simulink model "gm_wlanhdlTimeAndFrequencySynchronization"  (R2025a)
settings: Solver=FixedStepDiscrete  StartTime=0.0  StopTime=stopTime  RelTol=1e-3
InitFcn:
  | wlanFrontEndInit;
undefined symbols (not defined in the file or in its folder): a, b, c, Hd, wlanConfig
libraries: simulink x95, hdlsllib x16, hdlmdlgenlib x12, dspsrcs4 x3, dspsigops x3, dsphdlsigops2 x2, dsphdlfiltering2 x2
(part 1 of 11)
settings Model: Creator=The MathWorks, Inc.  LastModifiedBy=amd
settings SolverCC: MaxZcPerStep=1.0
settings OptimizationCC: BlockReduction=off  ConditionallyExecuteInputs=off  DefaultParameterBehavior=Inlined  ReuseModelBlockBuffer=off
settings DebuggingCC: AlgebraicLoopMsg=error  SaveWithParameterizedLinksMsg=none  InheritedTsInSrcMsg=none  SingleTaskRateTransMsg=error  UnconnectedInputMsg=warning  UnconnectedOutputMsg=warning  UnconnectedLineMsg=warning
settings HardwareCC: ProdBitPerPointer=32.0  ProdBitPerSizeT=32.0  ProdBitPerPtrDiffT=32.0  ProdLargestAtomicFloat=None  ProdIntDivRoundTo=Undefined  ProdEndianess=Unspecified  ProdWordSize=32.0  ProdHWDeviceType=ASIC/FPGA->ASIC/FPGA  TargetBitPerLong=64.0  TargetBitPerPointer=64.0  TargetBitPerSizeT=64.0  TargetBitPerPtrDiffT=64.0  TargetLongLongMode=on  TargetIntDivRoundTo=Zero  TargetEndianess=LittleEndian  TargetWordSize=64.0  TargetHWDeviceType=Custom Processor->MATLAB Host Computer  ProdEqTarget=off
settings ModelReferenceCC: EnableRefExpFcnMdlSchedulingChecks=on
settings RTWCC: GPUComputeCapability=3.5  DLArmComputeVersion=19.05

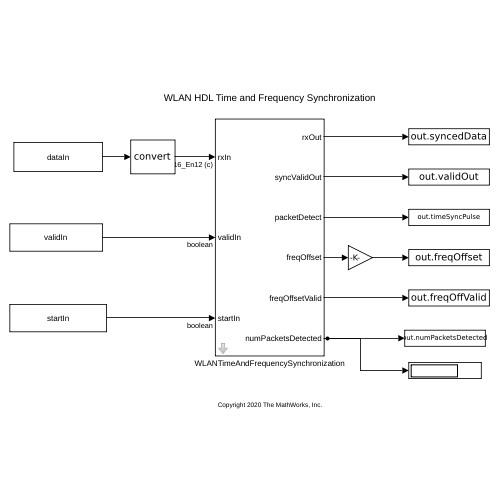
[thumbnail: Simulink's stored preview of the top-level diagram]
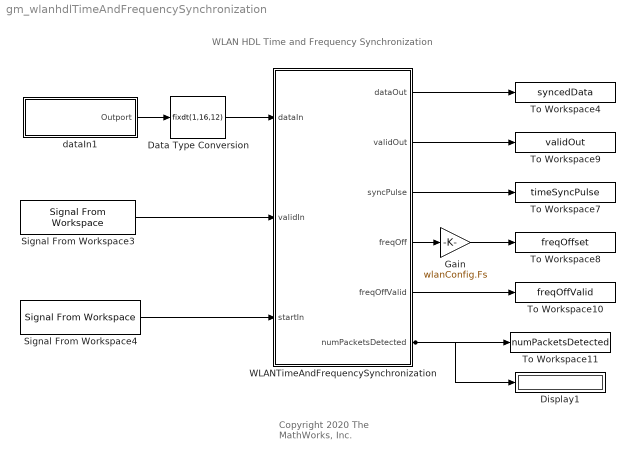
== system gm_wlanhdlTimeAndFrequencySynchronization ==
  note: WLAN HDL Time and Frequency Synchronization
  note: Copyright 2020 The MathWorks, Inc.
  Data Type Conversion : DataTypeConversion  OutDataTypeStr=fixdt(1,16,12)  SaturateOnIntegerOverflow=off  RndMeth=Floor
  Display1 : Display
  Gain : Gain  Gain=wlanConfig.Fs
  Signal From Workspace3 : dspsrcs4/Signal From Workspace  X=validIn  Ts=1/wlanConfig.Fs  nsamps=1  OutputAfterFinalValue=Setting to zero  ignoreOrWarnInputAndFrameLengths=off  OutputFrames=off
  Signal From Workspace4 : dspsrcs4/Signal From Workspace  X=startIn  Ts=1/wlanConfig.Fs  nsamps=1  OutputAfterFinalValue=Setting to zero  ignoreOrWarnInputAndFrameLengths=off  OutputFrames=off
  To Workspace10 : ToWorkspace  VariableName=freqOffValid  SampleTime=-1
      settings: Save2DSignal=2-D array (concatenate along first dimension)
  To Workspace11 : ToWorkspace  VariableName=numPacketsDetected  SampleTime=-1
      settings: Save2DSignal=2-D array (concatenate along first dimension)
  To Workspace4 : ToWorkspace  VariableName=syncedData  SampleTime=-1
      settings: Save2DSignal=2-D array (concatenate along first dimension)
  To Workspace7 : ToWorkspace  VariableName=timeSyncPulse  SampleTime=-1
      settings: Save2DSignal=2-D array (concatenate along first dimension)
  To Workspace8 : ToWorkspace  VariableName=freqOffset  SampleTime=-1
      settings: Save2DSignal=2-D array (concatenate along first dimension)
  To Workspace9 : ToWorkspace  VariableName=validOut  SampleTime=-1
      settings: Save2DSignal=2-D array (concatenate along first dimension)
  WLANTimeAndFrequencySynchronization : Subsystem  mask(WLAN Front end application){chanBW=20MHz}
      mask prompts: chanBW "Channel bandwidth:"
      mask help: Performs time and frequency synchronization.
      mask Help: eval('showExample(''whdl/WLANHDLTimeAndFrequencySynchronizationExample'')')
      mask TypeOptions chanBW: 20MHz | 40MHz | 80MHz
      mask Display:
      | port_label('input',1,'rxIn');
      | port_label('input',2,'validIn');
      | port_label('input',3,'startIn');
      | port_label('output',1,'rxOut');
      | port_label('output',2,'syncValidOut');
      | port_label('output',3,'packetDetect');
      | port_label('output',4,'freqOffset');
      | port_label('output',5,'freqOffsetValid');
      | 
      | port_label('output',6,'numPacketsDetected');
  dataIn1 : Subsystem
      mask Display: disp('dataIn');
  wires:
  Gain/1 -> To Workspace8/1
  WLANTimeAndFrequencySynchronization/4(freqOff) -> Gain/1
  dataIn1/1(Outport) -> Data Type Conversion/1
  Data Type Conversion/1 -> WLANTimeAndFrequencySynchronization/1(dataIn)
  WLANTimeAndFrequencySynchronization/1(dataOut) -> To Workspace4/1
  WLANTimeAndFrequencySynchronization/2(validOut) -> To Workspace9/1
  Signal From Workspace4/1 -> WLANTimeAndFrequencySynchronization/3(startIn)
  WLANTimeAndFrequencySynchronization/3(syncPulse) -> To Workspace7/1
  WLANTimeAndFrequencySynchronization/6(numPacketsDetected) -> Display1/1, To Workspace11/1
  WLANTimeAndFrequencySynchronization/5(freqOffValid) -> To Workspace10/1
  Signal From Workspace3/1 -> WLANTimeAndFrequencySynchronization/2(validIn)

== system gm_wlanhdlTimeAndFrequencySynchronization/WLANTimeAndFrequencySynchronization ==
  dataIn : Inport  OutDataTypeStr=fixdt(1, 16, 12)  PortDimensions=1  SampleTime=5e-08
      settings: SignalType=complex
  validIn : Inport  Port=2  OutDataTypeStr=boolean  PortDimensions=1  SampleTime=5e-08
  startIn : Inport  Port=3  OutDataTypeStr=boolean  PortDimensions=1  SampleTime=5e-08
  Add : Sum  OutDataTypeStr=fixdt(1, 35, 33)  AccumDataTypeStr=fixdt(1, 35, 33)  SampleTime=6.25e-09
  Coarse CFO Estimation and Correction : Subsystem
  Coarse Time Sync : Subsystem
  Delay1 : Delay  DelayLength=double(1)  InitialCondition=0  SampleTime=5e-08
  Delay2 : Delay  DelayLength=double(1)  InitialCondition=0  SampleTime=5e-08
  Delay3 : Delay  DelayLength=double(1)  InitialCondition=0  SampleTime=5e-08
  Fine CFO Estimation and Correction : Subsystem
  Fine Time Sync : Subsystem
  HDL Counter : RateTransition  InitialCondition=double(0)  OutPortSampleTimeOpt=Multiple of input port sample time  OutPortSampleTimeMultiple=8
  HDL Counter_absorbed : Delay  DelayLength=0
  Rx Filter : Subsystem
  adder : Sum  OutDataTypeStr=uint16  AccumDataTypeStr=uint16  SampleTime=6.25e-09
  compare : simulink/Logic and Bit Operations/Compare To Constant  relop===  const="fi(0,0,16,0,\"hex\",\"ffff\")"  OutDataTypeStr=boolean
  countFrom : Constant  Value=0  VectorParams1D=off  OutDataTypeStr=uint16  SampleTime=6.25e-09
  crp_out_delay : Delay  DelayLength=double(1)  InitialCondition=0  SampleTime=6.25e-09
  in0_repeat : RateTransition  Integrity=off  Deterministic=off  OutPortSampleTimeOpt=Multiple of input port sample time  OutPortSampleTimeMultiple=1/8
  in1_repeat : RateTransition  Integrity=off  Deterministic=off  OutPortSampleTimeOpt=Multiple of input port sample time  OutPortSampleTimeMultiple=1/8
  in2_repeat : RateTransition  Integrity=off  Deterministic=off  OutPortSampleTimeOpt=Multiple of input port sample time  OutPortSampleTimeMultiple=1/8
  in3_repeat : RateTransition  Integrity=off  Deterministic=off  OutPortSampleTimeOpt=Multiple of input port sample time  OutPortSampleTimeMultiple=1/8
  rd_{0,3..5} (4 alike) : Delay  DelayLength=double(1)  InitialCondition=0  SampleTime=6.25e-09
  rd_1 : Delay  DelayLength=double(3)  InitialCondition=0  SampleTime=6.25e-09
  rd_2 : Delay  DelayLength=double(2)  InitialCondition=0  SampleTime=6.25e-09
  step_value : Constant  VectorParams1D=off  OutDataTypeStr=uint16  SampleTime=6.25e-09
  switch : Switch  Criteria=u2 ~= 0  Threshold="fi(0,0,1,0,\"hex\",\"0\")"  OutDataTypeStr=uint16  SampleTime=6.25e-09  SaturateOnIntegerOverflow=off  InputSameDT=off
  switchEnable : MultiPortSwitch  DataPortOrder=Zero-based contiguous  Inputs=2  DiagnosticForDefault=None  zeroidx=on  OutDataTypeStr=uint16  SampleTime=6.25e-09  SaturateOnIntegerOverflow=off  InputSameDT=off
  t : RateTransition  InitialCondition=double(0)  OutPortSampleTimeOpt=Multiple of input port sample time  OutPortSampleTimeMultiple=8
  dataOut : Outport  SampleTime=5e-08
  validOut : Outport  Port=2  SampleTime=5e-08
  syncPulse : Outport  Port=3  SampleTime=5e-08
  freqOff : Outport  Port=4  SampleTime=5e-08
  freqOffValid : Outport  Port=5  SampleTime=5e-08
  numPacketsDetected : Outport  Port=6  SampleTime=5e-08
  wires:
  rd_5/1 -> switchEnable/3
  countFrom/1 -> switch/1
  compare/1 -> rd_3/1
  in1_repeat/1 -> rd_0/1
  rd_4/1 -> switch/3
  step_value/1 -> adder/2
  HDL Counter/1 -> HDL Counter_absorbed/1
  crp_out_delay/1 -> HDL Counter/1
  switchEnable/1 -> crp_out_delay/1
  t/1 -> freqOff/1
  rd_1/1 -> switchEnable/1
  rd_2/1 -> switchEnable/2
  in0_repeat/1 -> rd_1/1
  Coarse Time Sync/4(rst) -> Coarse CFO Estimation and Correction/4(rstIn)
  HDL Counter_absorbed/1 -> in1_repeat/1, numPacketsDetected/1
  Rx Filter/2(validOut) -> Coarse Time Sync/2(validIn)
  rd_0/1 -> rd_2/1, compare/1, adder/1
  Coarse CFO Estimation and Correction/3(validOut) -> Fine Time Sync/2(validIn)
  Add/1 -> t/1
  Delay1/1 -> Rx Filter/3(startIn)
  in2_repeat/1 -> Add/1
  Delay2/1 -> Rx Filter/2(validIn)
  Rx Filter/3(startOut) -> Coarse Time Sync/3(startIn)
  startIn/1 -> Delay1/1
  Coarse CFO Estimation and Correction/4(lstfStartOut) -> Fine Time Sync/3(lstfStart)
  validIn/1 -> Delay2/1
  Coarse Time Sync/2(validOut) -> Coarse CFO Estimation and Correction/2(validIn)
  Fine CFO Estimation and Correction/5(lstfStartOut) -> in0_repeat/1, syncPulse/1
  adder/1 -> rd_4/1
  Rx Filter/1(dataOut) -> Coarse Time Sync/1(dataIn)
  in3_repeat/1 -> Add/2
  Delay3/1 -> Rx Filter/1(dataIn)
  Fine Time Sync/2(validOut) -> Fine CFO Estimation and Correction/2(validIn)
  Coarse Time Sync/3(lstfStart) -> Coarse CFO Estimation and Correction/3(LSTF_start)
  dataIn/1 -> Delay3/1
  Coarse CFO Estimation and Correction/1(Freq) -> in2_repeat/1
  Coarse CFO Estimation and Correction/2(dataOut) -> Fine Time Sync/1(dataIn)
  switch/1 -> rd_5/1
  rd_3/1 -> switch/2
  Coarse Time Sync/1(dataOut) -> Coarse CFO Estimation and Correction/1(dataIn)
  Coarse CFO Estimation and Correction/5(rstOut) -> Fine Time Sync/4(rstIn)
  Fine CFO Estimation and Correction/1(Freq) -> in3_repeat/1
  Fine Time Sync/3(Lstf_start) -> Fine CFO Estimation and Correction/3(LSTF_start)
  Fine CFO Estimation and Correction/2(freqValidOut) -> freqOffValid/1
  Fine Time Sync/4(rstOut) -> Fine CFO Estimation and Correction/4(rstIn)
  Fine Time Sync/1(dataOut) -> Fine CFO Estimation and Correction/1(dataIn)
  Fine CFO Estimation and Correction/3(dataOut) -> dataOut/1
  Fine CFO Estimation and Correction/4(validOut) -> validOut/1

== system gm_wlanhdlTimeAndFrequencySynchronization/dataIn1 ==
  Signal From Workspace : dspsrcs4/Signal From Workspace  X=inputWaveform  Ts=1/wlanConfig.Fs  nsamps=1  OutputAfterFinalValue=Setting to zero  ignoreOrWarnInputAndFrameLengths=off  OutputFrames=off
  Outport : Outport
  wires:
  Signal From Workspace/1 -> Outport/1

== system gm_wlanhdlTimeAndFrequencySynchronization/WLANTimeAndFrequencySynchronization/Coarse CFO Estimation and Correction ==
  dataIn : Inport  OutDataTypeStr=fixdt(1, 16, 12)  PortDimensions=1  SampleTime=5e-08
      settings: SignalType=complex
  validIn : Inport  Port=2  OutDataTypeStr=boolean  PortDimensions=1  SampleTime=6.25e-09
  LSTF_start : Inport  Port=3  OutDataTypeStr=boolean  PortDimensions=1  SampleTime=6.25e-09
  rstIn : Inport  Port=4  OutDataTypeStr=boolean  PortDimensions=1  SampleTime=5e-08
  Coarse CFO Correction : Subsystem
  Coarse CFO Estimation : Subsystem
  Freq : Outport  SampleTime=5e-08
  dataOut : Outport  Port=2  SampleTime=5e-08
  validOut : Outport  Port=3  SampleTime=5e-08
  lstfStartOut : Outport  Port=4  SampleTime=5e-08
  rstOut : Outport  Port=5  SampleTime=5e-08
  wires:
  Coarse CFO Correction/5(rstOut) -> rstOut/1
  dataIn/1 -> Coarse CFO Estimation/1(dataIn)
  Coarse CFO Estimation/4(lstfStart) -> Coarse CFO Correction/4(lstfStartIn)
  validIn/1 -> Coarse CFO Estimation/2(validIn)
  rstIn/1 -> Coarse CFO Estimation/4(rstIn)
  Coarse CFO Correction/1(freqOut) -> Freq/1
  Coarse CFO Correction/2(dataOut) -> dataOut/1
  Coarse CFO Estimation/2(dataOut) -> Coarse CFO Correction/2(dataIn)
  Coarse CFO Estimation/3(validData) -> Coarse CFO Correction/3(validIn)
  LSTF_start/1 -> Coarse CFO Estimation/3(LSTF_start)
  Coarse CFO Correction/4(lstfStartOut) -> lstfStartOut/1
  Coarse CFO Estimation/5(rstOut) -> Coarse CFO Correction/5(rstIn)
  Coarse CFO Estimation/1(Freq) -> Coarse CFO Correction/1(freq)
  Coarse CFO Correction/3(validOut) -> validOut/1

== system gm_wlanhdlTimeAndFrequencySynchronization/WLANTimeAndFrequencySynchronization/Coarse Time Sync ==
  dataIn : Inport  OutDataTypeStr=fixdt(1, 16, 12)  PortDimensions=1  SampleTime=5e-08
      settings: SignalType=complex
  validIn : Inport  Port=2  OutDataTypeStr=boolean  PortDimensions=1  SampleTime=5e-08
  startIn : Inport  Port=3  OutDataTypeStr=boolean  PortDimensions=1  SampleTime=5e-08
  Correlator : Subsystem
  Delay4 : Delay  DelayLength=double(7)  InitialCondition=0  SampleTime=5e-08
  Delay6 : Delay  DelayLength=double(7)  InitialCondition=0  SampleTime=5e-08
  Energy Calculator : Subsystem
  Peak Detector : Subsystem
  Stream Synchronizer : Subsystem
  dataOut : Outport  SampleTime=5e-08  VectorParamsAs1DForOutWhenUnconnected=off
  validOut : Outport  Port=2  SampleTime=6.25e-09  VectorParamsAs1DForOutWhenUnconnected=off
  lstfStart : Outport  Port=3  SampleTime=6.25e-09  VectorParamsAs1DForOutWhenUnconnected=off
  rst : Outport  Port=4  SampleTime=5e-08  VectorParamsAs1DForOutWhenUnconnected=off
  wires:
  Peak Detector/2(validOut) -> validOut/1
  startIn/1 -> rst/1, Correlator/3(startIn)
  dataIn/1 -> Delay4/1, Energy Calculator/3(dataIn), Correlator/1(dataIn)
  validIn/1 -> Delay6/1, Correlator/2(validIn), Energy Calculator/4(validIn)
  Correlator/1(dataOut) -> Energy Calculator/1(corrIn)
  Correlator/2(validOut) -> Stream Synchronizer/1(corrValid), Energy Calculator/2(corrValidIn)
  Delay4/1 -> Stream Synchronizer/2(dataIn)
  Stream Synchronizer/1(dataOut) -> Peak Detector/4(dataIn)
  Peak Detector/1(lstfStart) -> lstfStart/1
  Delay6/1 -> Stream Synchronizer/3(dataValid)
  Peak Detector/3(dataOut) -> dataOut/1
  Energy Calculator/2(energyOut) -> Peak Detector/2(energyIn)
  Energy Calculator/3(validOut) -> Peak Detector/3(corrValid)
  Energy Calculator/1(corrOut) -> Peak Detector/1(corrIn)
  Stream Synchronizer/2(validOut) -> Peak Detector/5(dataValid)

== system gm_wlanhdlTimeAndFrequencySynchronization/WLANTimeAndFrequencySynchronization/Fine CFO Estimation and Correction ==
  dataIn : Inport  OutDataTypeStr=fixdt(1, 16, 12)  PortDimensions=1  SampleTime=5e-08
      settings: SignalType=complex
  validIn : Inport  Port=2  OutDataTypeStr=boolean  PortDimensions=1  SampleTime=6.25e-09
  LSTF_start : Inport  Port=3  OutDataTypeStr=boolean  PortDimensions=1  SampleTime=6.25e-09
  rstIn : Inport  Port=4  OutDataTypeStr=boolean  PortDimensions=1  SampleTime=5e-08
  Fine CFO Correction : Subsystem
  Fine CFO Estimation : Subsystem
  Freq : Outport  SampleTime=5e-08
  freqValidOut : Outport  Port=2  SampleTime=5e-08
  dataOut : Outport  Port=3  SampleTime=5e-08
  validOut : Outport  Port=4  SampleTime=5e-08
  lstfStartOut : Outport  Port=5  SampleTime=5e-08
  wires:
  dataIn/1 -> Fine CFO Estimation/1(dataIn)
  Fine CFO Correction/3(dataOut) -> dataOut/1
  validIn/1 -> Fine CFO Estimation/2(validIn)
  rstIn/1 -> Fine CFO Estimation/4(rstIn)
  Fine CFO Correction/4(validOut) -> validOut/1
  Fine CFO Correction/5(lstfStartOut) -> lstfStartOut/1
  LSTF_start/1 -> Fine CFO Estimation/3(LSTF_start)
  Fine CFO Estimation/1(Freq) -> Fine CFO Correction/1(freqIn)
  Fine CFO Estimation/3(dataOut) -> Fine CFO Correction/3(dataIn)
  Fine CFO Estimation/4(validOut) -> Fine CFO Correction/4(validIn)
  Fine CFO Correction/1(freqOut) -> Freq/1
  Fine CFO Estimation/2(freqValidOut) -> Fine CFO Correction/2(freqValidIn)
  Fine CFO Estimation/5(lstfStart) -> Fine CFO Correction/5(lstfStartIn)
  Fine CFO Correction/2(freqValidOut) -> freqValidOut/1

== system gm_wlanhdlTimeAndFrequencySynchronization/WLANTimeAndFrequencySynchronization/Fine Time Sync ==
  dataIn : Inport  OutDataTypeStr=fixdt(1, 16, 12)  PortDimensions=1  SampleTime=5e-08
      settings: SignalType=complex
  validIn : Inport  Port=2  OutDataTypeStr=boolean  PortDimensions=1  SampleTime=5e-08
  lstfStart : Inport  Port=3  OutDataTypeStr=boolean  PortDimensions=1  SampleTime=5e-08
  rstIn : Inport  Port=4  OutDataTypeStr=boolean  PortDimensions=1  SampleTime=5e-08
  Correlator : Subsystem
  Peak Searcher : Subsystem
  dataOut : Outport  SampleTime=5e-08  VectorParamsAs1DForOutWhenUnconnected=off
  validOut : Outport  Port=2  SampleTime=6.25e-09  VectorParamsAs1DForOutWhenUnconnected=off
  Lstf_start : Outport  Port=3  SampleTime=6.25e-09  VectorParamsAs1DForOutWhenUnconnected=off
  rstOut : Outport  Port=4  SampleTime=5e-08  VectorParamsAs1DForOutWhenUnconnected=off
  wires:
  Correlator/5(validOut) -> Peak Searcher/5(validIn)
  Correlator/3(startOut) -> Peak Searcher/3(startIn)
  Correlator/2(corrValid) -> Peak Searcher/2(corrValid)
  Peak Searcher/2(validOut) -> validOut/1
  Correlator/4(dataOut) -> Peak Searcher/4(dataIn)
  Correlator/1(corrOut) -> Peak Searcher/1(corrIn)
  rstIn/1 -> rstOut/1, Correlator/4(rstIn), Peak Searcher/6(rstIn)
  Peak Searcher/1(lstfStart) -> Lstf_start/1
  lstfStart/1 -> Correlator/3(startIn)
  validIn/1 -> Correlator/2(validIn)
  Peak Searcher/3(dataOut) -> dataOut/1
  dataIn/1 -> Correlator/1(dataIn)

== system gm_wlanhdlTimeAndFrequencySynchronization/WLANTimeAndFrequencySynchronization/Rx Filter ==
  dataIn : Inport  OutDataTypeStr=fixdt(1, 16, 12)  PortDimensions=1  SampleTime=5e-08
      settings: SignalType=complex
  validIn : Inport  Port=2  OutDataTypeStr=boolean  PortDimensions=1  SampleTime=5e-08
  startIn : Inport  Port=3  OutDataTypeStr=boolean  PortDimensions=1  SampleTime=5e-08
  DTConverter : Subsystem
  Delay : Delay  DelayLength=double(33)  InitialCondition=0  SampleTime=5e-08
  Discrete FIR Filter : dsphdlfiltering2/Discrete FIR Filter  NumeratorSource=Property  Numerator=Hd.Numerator  NumeratorPrototype=[]  FilterStructure=Direct form systolic  SerializationOption=Minimum number of cycles between valid input samples  NumCycles=2  NumberOfMultipliers=2  SimulateUsing=Code generation  roundingMode=Floor  overflowMode=off  CoefficientsDataTypeStr=Inherit: Same word length as input  OutputDataTypeStr=Inherit: Same word length as input  ResetInputPort=on  HDLGlobalReset=off  CoeffMultiplier=Multiplier  UseMultForPow2Coeff=on  FrameInputSymmOptim=off
  dataOut : Outport  SampleTime=5e-08
  validOut : Outport  Port=2  SampleTime=5e-08
  startOut : Outport  Port=3  SampleTime=5e-08
  wires:
  DTConverter/1(dataOut) -> dataOut/1
  Delay/1 -> startOut/1
  Discrete FIR Filter/2 -> validOut/1
  startIn/1 -> Discrete FIR Filter/3, Delay/1
  validIn/1 -> Discrete FIR Filter/2
  Discrete FIR Filter/1 -> DTConverter/2(dataIn2)
  dataIn/1 -> Discrete FIR Filter/1, DTConverter/1(dataIn1)

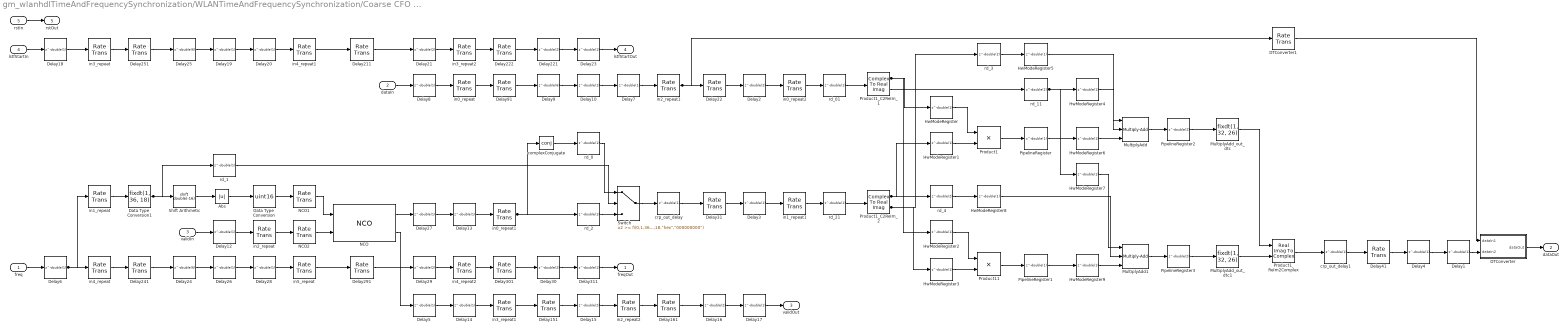
== system gm_wlanhdlTimeAndFrequencySynchronization/WLANTimeAndFrequencySynchronization/Coarse CFO Estimation and Correction/Coarse CFO Correction ==
  freq : Inport  OutDataTypeStr=fixdt(1, 34, 33)  PortDimensions=1  SampleTime=5e-08
  dataIn : Inport  Port=2  OutDataTypeStr=fixdt(1, 16, 12)  PortDimensions=1  SampleTime=5e-08
      settings: SignalType=complex
  validIn : Inport  Port=3  OutDataTypeStr=boolean  PortDimensions=1  SampleTime=5e-08
  lstfStartIn : Inport  Port=4  OutDataTypeStr=boolean  PortDimensions=1  SampleTime=5e-08
  rstIn : Inport  Port=5  OutDataTypeStr=boolean  PortDimensions=1  SampleTime=5e-08
  Abs : Abs  SampleTime=6.25e-09  OutDataTypeStr=fixdt(1, 36, 18)  SaturateOnIntegerOverflow=off
  DTConverter : Subsystem
  DTConverter1 : RateTransition  InitialCondition=double(0)  OutPortSampleTimeOpt=Multiple of input port sample time  OutPortSampleTimeMultiple=8
  Data Type  Conversion : DataTypeConversion  OutDataTypeStr=uint16  RndMeth=Round  SampleTime=6.25e-09  SaturateOnIntegerOverflow=off
  Data Type  Conversion1 : DataTypeConversion  OutDataTypeStr=fixdt(1, 36, 18)  SampleTime=6.25e-09  SaturateOnIntegerOverflow=off  RndMeth=Floor
  Delay{1,3..8,10,12..14,17..20,23,26..28,311} (20 alike) : Delay  DelayLength=double(1)  InitialCondition=0  SampleTime=5e-08
  Delay{2,15..16,21,29..30,221} (7 alike) : Delay  DelayLength=double(2)  InitialCondition=0  SampleTime=5e-08
  Delay{22,31,41,91,151,161,211,222,241,251,291,301} (12 alike) : RateTransition  InitialCondition=double(0)  OutPortSampleTimeOpt=Multiple of input port sample time  OutPortSampleTimeMultiple=8
  Delay24 : Delay  DelayLength=double(6)  InitialCondition=0  SampleTime=5e-08
  Delay25 : Delay  DelayLength=double(6)  InitialCondition=0  SampleTime=5e-08
  Delay9 : Delay  DelayLength=double(6)  InitialCondition=0  SampleTime=5e-08
  HwModeRegister{,1..9} (10 alike) : Delay  DelayLength=double(1)  InitialCondition=0  SampleTime=6.25e-09
  MultiplyAdd : hdlsllib/HDL Operations/Multiply-Add  Function=c-(a.*b)  datatype=fixdt(1, 33, 26)  DoSatur=off  FMA=off
  MultiplyAdd1 : hdlsllib/HDL Operations/Multiply-Add  Function=c+(a.*b)  datatype=fixdt(1, 33, 26)  DoSatur=off  FMA=off
  MultiplyAdd_out_dtc : DataTypeConversion  OutDataTypeStr=fixdt(1, 32, 26)  SampleTime=6.25e-09  SaturateOnIntegerOverflow=off  RndMeth=Floor
  MultiplyAdd_out_dtc1 : DataTypeConversion  OutDataTypeStr=fixdt(1, 32, 26)  SampleTime=6.25e-09  SaturateOnIntegerOverflow=off  RndMeth=Floor
  NCO : dsphdlsigops2/NCO  PhaseIncrementSource=Input port  PhaseIncrement=100  PhaseOffsetSource=Property  PhaseOffset=0  DitherSource=None  NumDitherBits=4  SamplesPerFrame=1  LUTCompress=off  ResetAction=off  Waveform=Complex exponential  PhasePort=off  SimulateUsing=Code generation  AccumulatorWL=16  PhaseQuantization=on  NumQuantizerAccumulatorBits=16  OutputDataType=Binary point scaling  OutputWL=16  OutputFL=14
  NCO1 : RateTransition  InitialCondition=double(0)  OutPortSampleTimeOpt=Multiple of input port sample time  OutPortSampleTimeMultiple=8
  NCO2 : RateTransition  InitialCondition=double(0)  OutPortSampleTimeOpt=Multiple of input port sample time  OutPortSampleTimeMultiple=8
  PipelineRegister : Delay  DelayLength=double(1)  InitialCondition=0  SampleTime=6.25e-09
  PipelineRegister1 : Delay  DelayLength=double(1)  InitialCondition=0  SampleTime=6.25e-09
  PipelineRegister2 : Delay  DelayLength=double(2)  InitialCondition=0  SampleTime=6.25e-09
  PipelineRegister3 : Delay  DelayLength=double(2)  InitialCondition=0  SampleTime=6.25e-09
  Product1 : Product  Inputs=**  OutDataTypeStr=fixdt(1, 32, 26)  SampleTime=6.25e-09
  Product11 : Product  Inputs=**  OutDataTypeStr=fixdt(1, 32, 26)  SampleTime=6.25e-09
  Product1_C2ReIm_1 : ComplexToRealImag  SampleTime=6.25e-09
  Product1_C2ReIm_2 : ComplexToRealImag  SampleTime=6.25e-09
  Product1_ReIm2Complex : RealImagToComplex  SampleTime=6.25e-09
  Shift Arithmetic : ArithShift  BitShiftNumber=double(-16)  BinPtShiftNumber=double(0)
  Switch : Switch  Threshold="fi(0,1,36,18,\"hex\",\"000000000\")"  OutDataTypeStr=fixdt(1, 16, 14)  SampleTime=6.25e-09  SaturateOnIntegerOverflow=off  InputSameDT=off
  complexConjugate : Math  Operator=conj  SignedPower=on  OutDataTypeStr=fixdt(1, 16, 14)
  crp_out_delay : Delay  DelayLength=double(1)  InitialCondition=0  SampleTime=6.25e-09
  crp_out_delay1 : Delay  DelayLength=double(1)  InitialCondition=0  SampleTime=6.25e-09
  in0_repeat : RateTransition  Integrity=off  Deterministic=off  OutPortSampleTimeOpt=Multiple of input port sample time  OutPortSampleTimeMultiple=1/8
  in0_repeat1 : RateTransition  Integrity=off  Deterministic=off  OutPortSampleTimeOpt=Multiple of input port sample time  OutPortSampleTimeMultiple=1/8
  in0_repeat2 : RateTransition  Integrity=off  Deterministic=off  OutPortSampleTimeOpt=Multiple of input port sample time  OutPortSampleTimeMultiple=1/8
  in1_repeat : RateTransition  Integrity=off  Deterministic=off  OutPortSampleTimeOpt=Multiple of input port sample time  OutPortSampleTimeMultiple=1/8
  in1_repeat1 : RateTransition  Integrity=off  Deterministic=off  OutPortSampleTimeOpt=Multiple of input port sample time  OutPortSampleTimeMultiple=1/8
  in2_repeat : RateTransition  Integrity=off  Deterministic=off  OutPortSampleTimeOpt=Multiple of input port sample time  OutPortSampleTimeMultiple=1/8
  in2_repeat1 : RateTransition  Integrity=off  Deterministic=off  OutPortSampleTimeOpt=Multiple of input port sample time  OutPortSampleTimeMultiple=1/8
  in2_repeat2 : RateTransition  Integrity=off  Deterministic=off  OutPortSampleTimeOpt=Multiple of input port sample time  OutPortSampleTimeMultiple=1/8
  in3_repeat : RateTransition  Integrity=off  Deterministic=off  OutPortSampleTimeOpt=Multiple of input port sample time  OutPortSampleTimeMultiple=1/8
  in3_repeat1 : RateTransition  Integrity=off  Deterministic=off  OutPortSampleTimeOpt=Multiple of input port sample time  OutPortSampleTimeMultiple=1/8
  in3_repeat2 : RateTransition  Integrity=off  Deterministic=off  OutPortSampleTimeOpt=Multiple of input port sample time  OutPortSampleTimeMultiple=1/8
  in4_repeat : RateTransition  Integrity=off  Deterministic=off  OutPortSampleTimeOpt=Multiple of input port sample time  OutPortSampleTimeMultiple=1/8
  in4_repeat1 : RateTransition  Integrity=off  Deterministic=off  OutPortSampleTimeOpt=Multiple of input port sample time  OutPortSampleTimeMultiple=1/8
  in4_repeat2 : RateTransition  Integrity=off  Deterministic=off  OutPortSampleTimeOpt=Multiple of input port sample time  OutPortSampleTimeMultiple=1/8
  in5_repeat : RateTransition  Integrity=off  Deterministic=off  OutPortSampleTimeOpt=Multiple of input port sample time  OutPortSampleTimeMultiple=1/8
  rd_{0..2,21} (4 alike) : Delay  DelayLength=double(1)  InitialCondition=0  SampleTime=6.25e-09
  rd_01 : Delay  DelayLength=double(1)  InitialCondition=0  SampleTime=6.25e-09
  rd_11 : Delay  DelayLength=double(2)  InitialCondition=0  SampleTime=6.25e-09
  rd_3 : Delay  DelayLength=double(2)  InitialCondition=0  SampleTime=6.25e-09
  rd_4 : Delay  DelayLength=double(2)  InitialCondition=0  SampleTime=6.25e-09
  freqOut : Outport  SampleTime=5e-08  VectorParamsAs1DForOutWhenUnconnected=off
  dataOut : Outport  Port=2  SampleTime=5e-08  VectorParamsAs1DForOutWhenUnconnected=off
  validOut : Outport  Port=3  SampleTime=5e-08  VectorParamsAs1DForOutWhenUnconnected=off
  lstfStartOut : Outport  Port=4  SampleTime=5e-08  VectorParamsAs1DForOutWhenUnconnected=off
  rstOut : Outport  Port=5  SampleTime=5e-08  VectorParamsAs1DForOutWhenUnconnected=off
  wires:
  DTConverter/1(dataOut) -> dataOut/1
  Delay41/1 -> Delay4/1
  Product1_ReIm2Complex/1 -> crp_out_delay1/1
  PipelineRegister3/1 -> MultiplyAdd_out_dtc1/1
  PipelineRegister2/1 -> MultiplyAdd_out_dtc/1
  MultiplyAdd1/1 -> PipelineRegister3/1
  MultiplyAdd/1 -> PipelineRegister2/1
  HwModeRegister4/1 -> MultiplyAdd/1
  PipelineRegister1/1 -> HwModeRegister9/1
  rd_11/1 -> HwModeRegister7/1, HwModeRegister4/1
  HwModeRegister5/1 -> MultiplyAdd/2
  HwModeRegister8/1 -> MultiplyAdd1/2
  Product1/1 -> PipelineRegister/1
  HwModeRegister2/1 -> Product11/1
  HwModeRegister1/1 -> Product1/2
  Product1_C2ReIm_2/1 -> HwModeRegister1/1, rd_4/1
  MultiplyAdd_out_dtc/1 -> Product1_ReIm2Complex/1
  Product1_C2ReIm_1/2 -> rd_11/1
  rd_21/1 -> Product1_C2ReIm_2/1
  rd_01/1 -> Product1_C2ReIm_1/1
  Delay17/1 -> validOut/1
  Delay3/1 -> in1_repeat1/1
  Delay2/1 -> in0_repeat2/1
  Delay16/1 -> Delay17/1
  Delay31/1 -> Delay3/1
  HwModeRegister/1 -> Product1/1
  Product1_C2ReIm_2/2 -> HwModeRegister3/1, rd_3/1
  crp_out_delay/1 -> Delay31/1
  Product11/1 -> PipelineRegister1/1
  in2_repeat1/1 -> Delay22/1, DTConverter1/1
  crp_out_delay1/1 -> Delay41/1
  Switch/1 -> crp_out_delay/1
  Delay211/1 -> Delay21/1
  Delay22/1 -> Delay2/1
  in3_repeat/1 -> Delay251/1
  Delay28/1 -> in5_repeat/1
  Delay12/1 -> in2_repeat/1
  rd_1/1 -> Switch/2
  Delay251/1 -> Delay25/1
  Data Type  Conversion1/1 -> Shift Arithmetic/1, rd_1/1
  in2_repeat2/1 -> Delay161/1
  Delay311/1 -> freqOut/1
  NCO1/1 -> NCO/1
  in2_repeat/1 -> NCO2/1
  DTConverter1/1 -> DTConverter/1(dataIn1)
  Delay19/1 -> Delay20/1
  in1_repeat1/1 -> rd_21/1
  in0_repeat2/1 -> rd_01/1
  Abs/1 -> Data Type  Conversion/1
  Delay24/1 -> Delay26/1
  rd_3/1 -> HwModeRegister5/1
  Delay20/1 -> in4_repeat1/1
  in1_repeat/1 -> Data Type  Conversion1/1
  validIn/1 -> Delay12/1
  rstIn/1 -> rstOut/1
  HwModeRegister3/1 -> Product11/2
  in3_repeat2/1 -> Delay222/1
  Delay27/1 -> Delay13/1
  lstfStartIn/1 -> Delay18/1
  Delay30/1 -> Delay311/1
  Shift Arithmetic/1 -> Abs/1
  Delay18/1 -> in3_repeat/1
  Delay7/1 -> in2_repeat1/1
  Delay6/1 -> in4_repeat/1, in1_repeat/1
  Delay29/1 -> in4_repeat2/1
  NCO2/1 -> NCO/2
  Delay161/1 -> Delay16/1
  freq/1 -> Delay6/1
  Delay25/1 -> Delay19/1
  Delay9/1 -> Delay10/1
  Data Type  Conversion/1 -> NCO1/1
  in4_repeat/1 -> Delay241/1
  HwModeRegister6/1 -> MultiplyAdd/3
  in5_repeat/1 -> Delay291/1
  Delay241/1 -> Delay24/1
  HwModeRegister9/1 -> MultiplyAdd1/3
  dataIn/1 -> Delay8/1
  NCO/1 -> Delay27/1
  in3_repeat1/1 -> Delay151/1
  Delay1/1 -> DTConverter/2(dataIn2)
  NCO/2 -> Delay5/1
  MultiplyAdd_out_dtc1/1 -> Product1_ReIm2Complex/2
  Delay26/1 -> Delay28/1
  Delay221/1 -> Delay23/1
  PipelineRegister/1 -> HwModeRegister6/1
  Delay21/1 -> in3_repeat2/1
  Delay291/1 -> Delay29/1
  Delay8/1 -> in0_repeat/1
  complexConjugate/1 -> rd_0/1
  Delay5/1 -> Delay14/1
  in0_repeat/1 -> Delay91/1
  Delay13/1 -> in0_repeat1/1
  in4_repeat2/1 -> Delay301/1
  HwModeRegister7/1 -> MultiplyAdd1/1
  Delay14/1 -> in3_repeat1/1
  Delay222/1 -> Delay221/1
  Delay4/1 -> Delay1/1
  in0_repeat1/1 -> complexConjugate/1, rd_2/1
  Delay91/1 -> Delay9/1
  Delay301/1 -> Delay30/1
  Delay151/1 -> Delay15/1
  in4_repeat1/1 -> Delay211/1
  Delay10/1 -> Delay7/1
  rd_4/1 -> HwModeRegister8/1
  Product1_C2ReIm_1/1 -> HwModeRegister2/1, HwModeRegister/1
  Delay23/1 -> lstfStartOut/1
  rd_0/1 -> Switch/1
  rd_2/1 -> Switch/3
  Delay15/1 -> in2_repeat2/1
